simulink subsystem "SuspensionSystem"  (R2022a)
settings: Solver=VariableStepAuto  StartTime=0.0  StopTime=10.0  RelTol=1e-3
values from neighbouring files (symbols this model uses):
  c = 100    [SYDE351Project.m]
  k = 10000    [SYDE351Project.m]
  mass = 20    [SYDE351Project.m]
  mass_loaded = 40    [SYDE351Project.m]
settings Model: Creator=Bronz  LastModifiedBy=lanam

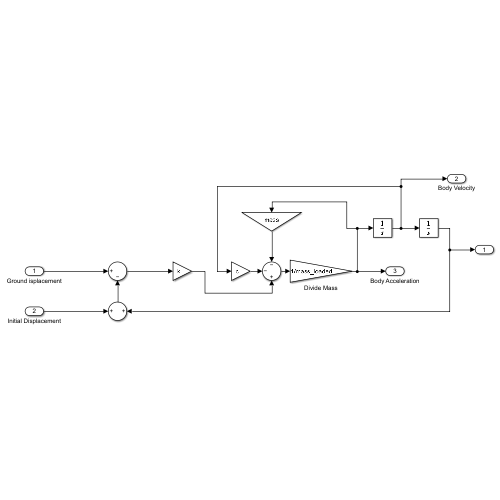
[thumbnail: Simulink's stored preview of the top-level diagram]
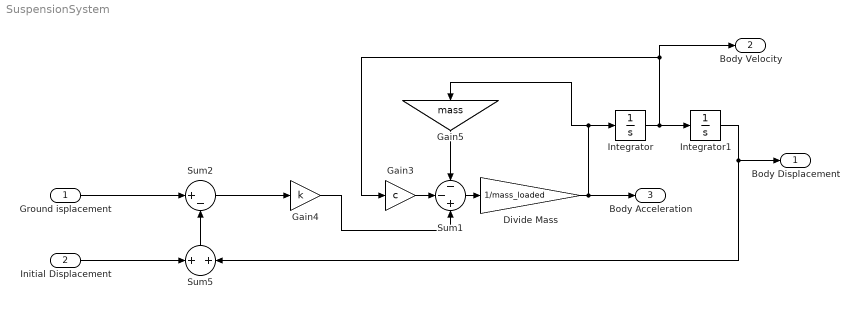
== system SuspensionSystem ==
  Ground isplacement : Inport
  Initial Displacement : Inport  Port=2
  Divide Mass : Gain  Gain=1/mass_loaded
  Gain3 : Gain  Gain=c
  Gain4 : Gain  Gain=k
  Gain5 : Gain  Gain=mass
  Integrator : Integrator
  Integrator1 : Integrator
  Sum1 : Sum  Inputs=--+
  Sum2 : Sum  Inputs=|+-
  Sum5 : Sum  Inputs=+|+
  Body Displacement : Outport
  Body Velocity : Outport  Port=2
  Body Acceleration : Outport  Port=3
  wires:
  Sum1/1 -> Divide Mass/1
  Ground isplacement/1 -> Sum2/1
  Integrator1/1 -> Sum5/2, Body Displacement/1
  Sum2/1 -> Gain4/1
  Sum5/1 -> Sum2/2
  Initial Displacement/1 -> Sum5/1
  Integrator/1 -> Body Velocity/1, Gain3/1, Integrator1/1
  Divide Mass/1 -> Gain5/1, Integrator/1, Body Acceleration/1
  Gain3/1 -> Sum1/2
  Gain5/1 -> Sum1/1
  Gain4/1 -> Sum1/3
